simulink model "bd_par_auto2"  (Simulink 4.1.1)
settings: Solver=ode1  SolverMode=SingleTasking  StartTime=0.0  StopTime=max(cyc_mph(:,1))  FixedStep=1  MaxStep=1  RelTol=1e-3  AbsTol=1e-3
undefined symbols (not defined in the file): air_cp, amb_tmp, cs_charge_deplete_bool, cs_charge_trq, cs_electric_decel_spd, cs_electric_launch_spd_hi, cs_electric_launch_spd_lo, cs_hi_soc, cs_lo_soc, cs_min_trq_frac, cs_off_trq_frac, cyc_avg_time, cyc_cargo_mass, cyc_elevation_init, cyc_filter_bool, cyc_grade, cyc_mph, enable_stop, ess_cap_scale, ess_coulombic_eff, ess_init_soc, ess_max_ah_cap, ess_max_volts, ess_min_volts, ess_mod_airflow, ess_mod_cp, ess_mod_init_tmp, ess_module_mass, ess_module_num, ess_on, ess_res_scale_coef, ess_res_scale_fun, ess_set_tmp, ess_th_calc, ess_th_res_off, ess_th_res_on, ess_tmp, ess_voc, ex_calc, fc_ct_trq, fc_emis, fc_inertia, fc_map_spd, fc_max_trq, fc_on, fc_spd_scale, fc_trq_scale, fc_tstat, fd_inertia, fd_loss, fd_ratio, gb_dnshift_load, gb_dnshift_spd, gb_gears_num, gb_inertia, gb_num_init, gb_ratio, gb_shift_delay, gb_spd_scale, gb_trq_scale ... (+56)
libraries: lib_wheel2 x12, lib_accessory2 x3, lib_etc x2, lib_drive_cycle2 x1, lib_interactive x1, lib_drive_cycle x1, lib_exhaust x1, lib_fuel_converter3 x1
(part 3 of 18)

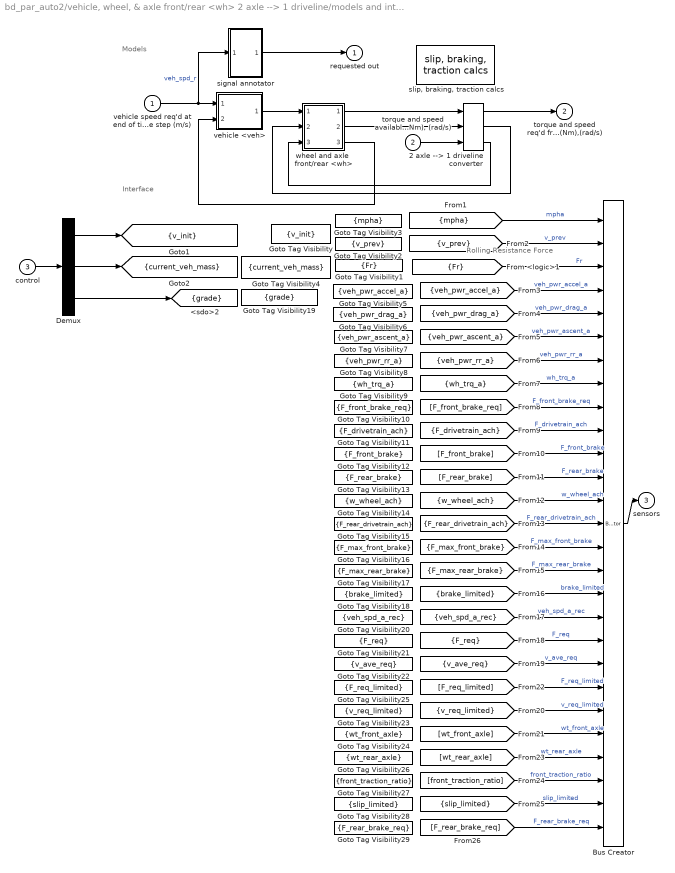
== system bd_par_auto2/vehicle, wheel, & axle front/rear <wh> 2 axle --> 1 driveline/models and interface ==
  note: Interface
  note: Models
  note: Rolling Resistance Force
  vehicle speed req'd at end of time step (m/s) : Inport  Port=1  LatchInput=off
  "torque and speed available from drivetrain into axles (Nm), (rad/s)" : Inport  Port=2  LatchInput=off
  control : Inport  Port=3  LatchInput=off
  2 axle --> 1 driveline converter : lib_wheel2/Submodels/2 axle --> 1 driveline converter
      settings: RTWFcnNameOpts=Auto  RTWFileNameOpts=Auto
  Bus Creator : BusCreator  Inputs=27
  Demux : Demux  Outputs=3  BusSelectionMode=off
  Goto Tag Visibility : GotoTagVisibility  GotoTag=v_init
  Goto Tag Visibility1 : GotoTagVisibility  GotoTag=Fr
  Goto Tag Visibility10 : GotoTagVisibility  GotoTag=F_front_brake_req
  Goto Tag Visibility11 : GotoTagVisibility  GotoTag=F_drivetrain_ach
  Goto Tag Visibility12 : GotoTagVisibility  GotoTag=F_front_brake
  Goto Tag Visibility13 : GotoTagVisibility  GotoTag=F_rear_brake
  Goto Tag Visibility14 : GotoTagVisibility  GotoTag=w_wheel_ach
  Goto Tag Visibility15 : GotoTagVisibility  GotoTag=F_rear_drivetrain_ach
  Goto Tag Visibility16 : GotoTagVisibility  GotoTag=F_max_front_brake
  Goto Tag Visibility17 : GotoTagVisibility  GotoTag=F_max_rear_brake
  Goto Tag Visibility18 : GotoTagVisibility  GotoTag=brake_limited
  Goto Tag Visibility19 : GotoTagVisibility  GotoTag=grade
  Goto Tag Visibility2 : GotoTagVisibility  GotoTag=v_prev
  Goto Tag Visibility20 : GotoTagVisibility  GotoTag=veh_spd_a_rec
  Goto Tag Visibility21 : GotoTagVisibility  GotoTag=F_req
  Goto Tag Visibility22 : GotoTagVisibility  GotoTag=v_ave_req
  Goto Tag Visibility23 : GotoTagVisibility  GotoTag=v_req_limited
  Goto Tag Visibility24 : GotoTagVisibility  GotoTag=wt_front_axle
  Goto Tag Visibility25 : GotoTagVisibility  GotoTag=F_req_limited
  Goto Tag Visibility26 : GotoTagVisibility  GotoTag=wt_rear_axle
  Goto Tag Visibility27 : GotoTagVisibility  GotoTag=front_traction_ratio
  Goto Tag Visibility28 : GotoTagVisibility  GotoTag=slip_limited
  Goto Tag Visibility29 : GotoTagVisibility  GotoTag=F_rear_brake_req
  Goto Tag Visibility3 : GotoTagVisibility  GotoTag=mpha
  Goto Tag Visibility4 : GotoTagVisibility  GotoTag=current_veh_mass
  Goto Tag Visibility5 : GotoTagVisibility  GotoTag=veh_pwr_accel_a
  Goto Tag Visibility6 : GotoTagVisibility  GotoTag=veh_pwr_drag_a
  Goto Tag Visibility7 : GotoTagVisibility  GotoTag=veh_pwr_ascent_a
  Goto Tag Visibility8 : GotoTagVisibility  GotoTag=veh_pwr_rr_a
  Goto Tag Visibility9 : GotoTagVisibility  GotoTag=wh_trq_a
  signal annotator : Subsystem
      settings: RTWFcnNameOpts=Auto  RTWFileNameOpts=Auto
  "slip, braking, traction calcs" : lib_wheel2/vehicle, wheel, & axle front//rear <wh>/models and interface/slip, braking, traction calcs
      link override config traction control: BlockChoice=traction control 2 axle
      settings: RTWFcnNameOpts=Auto  RTWFileNameOpts=Auto
  vehicle <veh> : Subsystem
      settings: RTWFcnNameOpts=Auto  RTWFileNameOpts=Auto
      mask Display: image(imread('bdi_veh.jpg'))
  wheel and axle  front/rear <wh> : Subsystem
      settings: RTWFcnNameOpts=Auto  RTWFileNameOpts=Auto
      mask Display: image(imread('bdi_wh.jpg'))
  requested out : Outport  Port=1  InitialOutput=0
  torque and speed req'd from drivetrain into axles (Nm),(rad/s) : Outport  Port=2  InitialOutput=0
  sensors : Outport  Port=3  InitialOutput=0
  tag scope: current_veh_mass=scoped, grade=scoped, v_init=scoped
  wires:
  signal annotator/1(Out1) -> requested out/1
  [F_rear_brake_req] -> Bus Creator/27  "F_rear_brake_req"
  [slip_limited] -> Bus Creator/26  "slip_limited"
  2 axle --> 1 driveline converter/1 -> torque and speed req'd from drivetrain into axles (Nm),(rad/s)/1
  2 axle --> 1 driveline converter/3 -> wheel and axle  front/rear <wh>/3("torque and speed available from drivetrain into rear axle (Nm), (rad/s)")
  2 axle --> 1 driveline converter/2 -> wheel and axle  front/rear <wh>/2("torque and speed available from drivetrain into front axle (Nm), (rad/s)")
  "torque and speed available from drivetrain into axles (Nm), (rad/s)"/1 -> 2 axle --> 1 driveline converter/3
  [front_traction_ratio] -> Bus Creator/25  "front_traction_ratio"
  [wt_rear_axle] -> Bus Creator/24  "wt_rear_axle"
  [wt_front_axle] -> Bus Creator/23  "wt_front_axle"
  [v_req_limited] -> Bus Creator/22  "v_req_limited"
  [F_req_limited] -> Bus Creator/21  "F_req_limited"
  [v_ave_req] -> Bus Creator/20  "v_ave_req"
  [F_req] -> Bus Creator/19  "F_req"
  [veh_spd_a_rec] -> Bus Creator/18  "veh_spd_a_rec"
  [brake_limited] -> Bus Creator/17  "brake_limited"
  [F_max_rear_brake] -> Bus Creator/16  "F_max_rear_brake"
  [F_max_front_brake] -> Bus Creator/15  "F_max_front_brake"
  [F_rear_drivetrain_ach] -> Bus Creator/14  "F_rear_drivetrain_ach"
  [w_wheel_ach] -> Bus Creator/13  "w_wheel_ach"
  [F_rear_brake] -> Bus Creator/12  "F_rear_brake"
  [F_front_brake] -> Bus Creator/11  "F_front_brake"
  [F_drivetrain_ach] -> Bus Creator/10  "F_drivetrain_ach"
  [F_front_brake_req] -> Bus Creator/9  "F_front_brake_req"
  [wh_trq_a] -> Bus Creator/8  "wh_trq_a"
  [veh_pwr_rr_a] -> Bus Creator/7  "veh_pwr_rr_a"
  [veh_pwr_ascent_a] -> Bus Creator/6  "veh_pwr_ascent_a"
  [veh_pwr_drag_a] -> Bus Creator/5  "veh_pwr_drag_a"
  [veh_pwr_accel_a] -> Bus Creator/4  "veh_pwr_accel_a"
  [v_prev] -> Bus Creator/2  "v_prev"
  [mpha] -> Bus Creator/1  "mpha"
  Bus Creator/1 -> sensors/1
  [Fr] -> Bus Creator/3  "Fr"
  Demux/3 -> [grade]
  Demux/2 -> [current_veh_mass]
  Demux/1 -> [v_init]
  control/1 -> Demux/1
  wheel and axle  front/rear <wh>/2(torque and speed req'd from drivetrain into rear axle (Nm),(rad/s)) -> 2 axle --> 1 driveline converter/2
  wheel and axle  front/rear <wh>/1(torque and speed req'd from drivetrain into front axle (Nm),(rad/s)) -> 2 axle --> 1 driveline converter/1
  wheel and axle  front/rear <wh>/3(tractive force and linear speed  achievable) -> vehicle <veh>/2(tractive force and linear speed achievable (N))
  vehicle <veh>/1("tractive force and speed required of tire and wheel (N), (m/s)") -> wheel and axle  front/rear <wh>/1("tractive force and speed req'd of tire/road interface (N), (m/s)")
  vehicle speed req'd at end of time step (m/s)/1 -> vehicle <veh>/1(vehicle speed req'd at end of time step (m/s)), signal annotator/1(veh_spd_r)  "veh_spd_r"

== system bd_par_auto2/<cs> control strategy/Automatic Transmission  Control/gearbox control for automatic transmission ==
  "eta_gb, t=(i-1)" : Inport  Port=1  LatchInput=off
  T_gb_out : Inport  Port=2  LatchInput=off
  w_gb_out : Inport  Port=3  LatchInput=off
  slip_limited : Inport  Port=4  LatchInput=off
  Goto Tag Visibility10 : GotoTagVisibility  GotoTag=gear_number
  Goto Tag Visibility11 : GotoTagVisibility  GotoTag=shifting
  Goto Tag Visibility12 : GotoTagVisibility  GotoTag=gear_ratio
  Goto Tag Visibility13 : GotoTagVisibility  GotoTag=locked_up
  Goto Tag Visibility6 : GotoTagVisibility  GotoTag=T_gb_out
  Goto Tag Visibility7 : GotoTagVisibility  GotoTag=w_gb_out
  Goto Tag Visibility8 : GotoTagVisibility  GotoTag=eta_gb
  Goto Tag Visibility9 : GotoTagVisibility  GotoTag=slip_limited
  gearbox control for use w/ AT : Subsystem
      settings: RTWFcnNameOpts=Auto  RTWFileNameOpts=Auto
  gear ratio : Outport  Port=1  InitialOutput=0
  shifting : Outport  Port=2  InitialOutput=0
  gear number : Outport  Port=3  InitialOutput=0
  locked_up : Outport  Port=4  InitialOutput=0
  tag scope: T_gb_out=scoped, eta_gb=scoped, gear_number=scoped, gear_ratio=scoped, locked_up=scoped, shifting=scoped, slip_limited=scoped, w_gb_out=scoped
  wires:
  T_gb_out/1 -> [T_gb_out]
  w_gb_out/1 -> [w_gb_out]
  [gear_number] -> gear number/1
  [shifting] -> shifting/1
  [gear_ratio] -> gear ratio/1
  slip_limited/1 -> [slip_limited]
  "eta_gb, t=(i-1)"/1 -> [eta_gb]
  [slip_limited] -> gearbox control for use w/ AT/4(tires are at traction limit)
  [w_gb_out] -> gearbox control for use w/ AT/3(gb_spd_out_r)
  [T_gb_out] -> gearbox control for use w/ AT/2(gb_trq_out_r)
  [eta_gb] -> gearbox control for use w/ AT/1(eta_gb)
  [locked_up] -> locked_up/1
  gearbox control for use w/ AT/1(gear ratio) -> [gear_ratio]
  gearbox control for use w/ AT/2(shifting) -> [shifting]
  gearbox control for use w/ AT/3(gear number) -> [gear_number]
  gearbox control for use w/ AT/4(locked up) -> [locked_up]

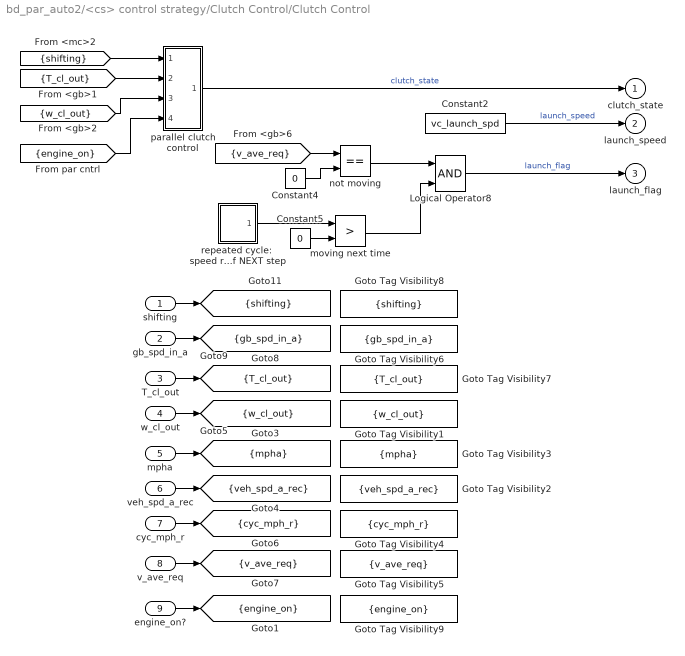
== system bd_par_auto2/<cs> control strategy/Clutch Control/Clutch Control ==
  shifting : Inport  Port=1  LatchInput=off
  gb_spd_in_a : Inport  Port=2  LatchInput=off
  T_cl_out : Inport  Port=3  LatchInput=off
  w_cl_out : Inport  Port=4  LatchInput=off
  mpha : Inport  Port=5  LatchInput=off
  veh_spd_a_rec : Inport  Port=6  LatchInput=off
  cyc_mph_r : Inport  Port=7  LatchInput=off
  v_ave_req : Inport  Port=8  LatchInput=off
  engine_on? : Inport  Port=9  LatchInput=off
  Constant2 : Constant  Value=vc_launch_spd
  Constant4 : Constant  Value=0
  Constant5 : Constant  Value=0
  Goto Tag Visibility1 : GotoTagVisibility  GotoTag=w_cl_out
  Goto Tag Visibility2 : GotoTagVisibility  GotoTag=veh_spd_a_rec
  Goto Tag Visibility3 : GotoTagVisibility  GotoTag=mpha
  Goto Tag Visibility4 : GotoTagVisibility  GotoTag=cyc_mph_r
  Goto Tag Visibility5 : GotoTagVisibility  GotoTag=v_ave_req
  Goto Tag Visibility6 : GotoTagVisibility  GotoTag=gb_spd_in_a
  Goto Tag Visibility7 : GotoTagVisibility  GotoTag=T_cl_out
  Goto Tag Visibility8 : GotoTagVisibility  GotoTag=shifting
  Goto Tag Visibility9 : GotoTagVisibility  GotoTag=engine_on
  Logical Operator8 : Logic  Operator=AND  Inputs=2
  moving next time : RelationalOperator  Operator=>
  not moving : RelationalOperator  Operator===
  parallel clutch control : Subsystem
      settings: RTWFcnNameOpts=Auto  RTWFileNameOpts=Auto
  repeated cycle:  speed required at end of NEXT step : Subsystem  mask(Forward looking repeating table){t=cyc_mph(:,1), y=cyc_mph(:,2)}
      mask prompts: t "Time values:"; y "Output values:"
      mask help:
      | Forward looking repeating table.
      | Enter values of time and output for first cycle.
      mask init:
      | period = max(t);
      settings: RTWFcnNameOpts=Auto  RTWFileNameOpts=Auto
      mask Help: Repeats cycle given in table with a one time step forward offset. Time values should be monotonically increasing.
  clutch_state : Outport  Port=1  InitialOutput=0
  launch_speed : Outport  Port=2  InitialOutput=0
  launch_flag : Outport  Port=3  InitialOutput=0
  tag scope: T_cl_out=scoped, cyc_mph_r=scoped, engine_on=scoped, gb_spd_in_a=scoped, mpha=scoped, shifting=scoped, v_ave_req=scoped, veh_spd_a_rec=scoped, w_cl_out=scoped
  wires:
  veh_spd_a_rec/1 -> [veh_spd_a_rec]
  T_cl_out/1 -> [T_cl_out]
  shifting/1 -> [shifting]
  gb_spd_in_a/1 -> [gb_spd_in_a]
  v_ave_req/1 -> [v_ave_req]
  cyc_mph_r/1 -> [cyc_mph_r]
  mpha/1 -> [mpha]
  w_cl_out/1 -> [w_cl_out]
  Constant2/1 -> launch_speed/1  "launch_speed"
  not moving/1 -> Logical Operator8/1
  Logical Operator8/1 -> launch_flag/1  "launch_flag"
  Constant4/1 -> not moving/2
  [v_ave_req] -> not moving/1
  repeated cycle:  speed required at end of NEXT step/1(out_1) -> moving next time/1
  Constant5/1 -> moving next time/2
  moving next time/1 -> Logical Operator8/2
  [engine_on] -> parallel clutch control/4(engine on)
  [T_cl_out] -> parallel clutch control/2(gb_trq_in_r)
  [w_cl_out] -> parallel clutch control/3(gb_spd_in_r)
  [shifting] -> parallel clutch control/1(shifting)
  parallel clutch control/1(clutch state) -> clutch_state/1  "clutch_state"
  engine_on?/1 -> [engine_on]

== system bd_par_auto2/<cs> control strategy/Electrical Accessories/electrical accessory controller ==
  electrical accessories on? : Inport  Port=1  LatchInput=off
  F_req in : Inport  Port=2  LatchInput=off
  key_on in : Inport  Port=3  LatchInput=off
  engine_on in : Inport  Port=4  LatchInput=off
  acc_on : Outport  Port=1  InitialOutput=0
  F_req : Outport  Port=2  InitialOutput=0
  key_on : Outport  Port=3  InitialOutput=0
  engine_on : Outport  Port=4  InitialOutput=0
  wires:
  electrical accessories on?/1 -> acc_on/1  "acc_on"
  engine_on in/1 -> engine_on/1  "engine_on"
  F_req in/1 -> F_req/1  "F_req"
  key_on in/1 -> key_on/1  "key_on"

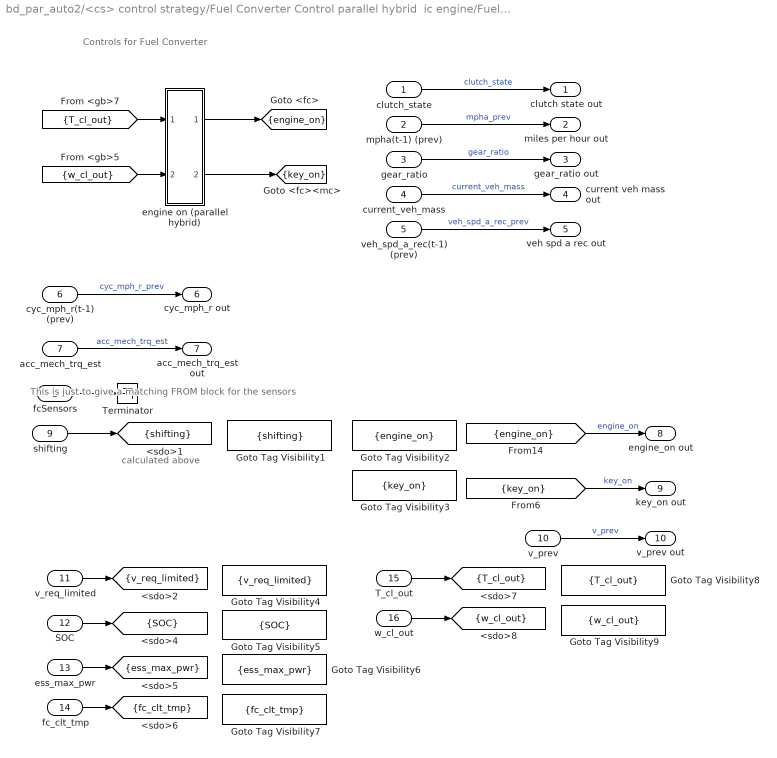
== system bd_par_auto2/<cs> control strategy/Fuel Converter Control parallel hybrid  ic engine/Fuel Converter Control ==
  note: Controls for Fuel Converter
  note: This is just to give a matching FROM block for the sensors
  note: calculated above
  clutch_state : Inport  Port=1  LatchInput=off
  mpha(t-1) (prev) : Inport  Port=2  LatchInput=off
  gear_ratio : Inport  Port=3  LatchInput=off
  current_veh_mass : Inport  Port=4  LatchInput=off
  veh_spd_a_rec(t-1) (prev) : Inport  Port=5  LatchInput=off
  cyc_mph_r(t-1) (prev) : Inport  Port=6  LatchInput=off
  acc_mech_trq_est : Inport  Port=7  LatchInput=off
  fcSensors : Inport  Port=8  LatchInput=off
  shifting : Inport  Port=9  LatchInput=off
  v_prev : Inport  Port=10  LatchInput=off
  v_req_limited : Inport  Port=11  LatchInput=off
  SOC : Inport  Port=12  LatchInput=off
  ess_max_pwr : Inport  Port=13  LatchInput=off
  fc_clt_tmp : Inport  Port=14  LatchInput=off
  T_cl_out : Inport  Port=15  LatchInput=off
  w_cl_out : Inport  Port=16  LatchInput=off
  Goto Tag Visibility1 : GotoTagVisibility  GotoTag=shifting
  Goto Tag Visibility2 : GotoTagVisibility  GotoTag=engine_on
  Goto Tag Visibility3 : GotoTagVisibility  GotoTag=key_on
  Goto Tag Visibility4 : GotoTagVisibility  GotoTag=v_req_limited
  Goto Tag Visibility5 : GotoTagVisibility  GotoTag=SOC
  Goto Tag Visibility6 : GotoTagVisibility  GotoTag=ess_max_pwr
  Goto Tag Visibility7 : GotoTagVisibility  GotoTag=fc_clt_tmp
  Goto Tag Visibility8 : GotoTagVisibility  GotoTag=T_cl_out
  Goto Tag Visibility9 : GotoTagVisibility  GotoTag=w_cl_out
  Terminator : Terminator
  engine on (parallel hybrid) : Subsystem
      settings: RTWFcnNameOpts=Auto  RTWFileNameOpts=Auto
  clutch state out : Outport  Port=1
  miles per hour out : Outport  Port=2
  gear_ratio out : Outport  Port=3
  current veh mass out : Outport  Port=4
  veh spd a rec out : Outport  Port=5
  cyc_mph_r out : Outport  Port=6
  acc_mech_trq_est out : Outport  Port=7
  engine_on out : Outport  Port=8
  key_on out : Outport  Port=9
  v_prev out : Outport  Port=10
  tag scope: SOC=scoped, T_cl_out=scoped, engine_on=scoped, ess_max_pwr=scoped, fc_clt_tmp=scoped, key_on=scoped, shifting=scoped, v_req_limited=scoped, w_cl_out=scoped
  wires:
  gear_ratio/1 -> gear_ratio out/1  "gear_ratio"
  fcSensors/1 -> Terminator/1
  shifting/1 -> [shifting]
  clutch_state/1 -> clutch state out/1  "clutch_state"
  mpha(t-1) (prev)/1 -> miles per hour out/1  "mpha_prev"
  current_veh_mass/1 -> current veh mass out/1  "current_veh_mass"
  veh_spd_a_rec(t-1) (prev)/1 -> veh spd a rec out/1  "veh_spd_a_rec_prev"
  cyc_mph_r(t-1) (prev)/1 -> cyc_mph_r out/1  "cyc_mph_r_prev"
  acc_mech_trq_est/1 -> acc_mech_trq_est out/1  "acc_mech_trq_est"
  v_prev/1 -> v_prev out/1  "v_prev"
  [engine_on] -> engine_on out/1  "engine_on"
  [key_on] -> key_on out/1  "key_on"
  engine on (parallel hybrid)/1(engine on) -> [engine_on]
  [T_cl_out] -> engine on (parallel hybrid)/1(trq req'd out of clutch (N*m))
  [w_cl_out] -> engine on (parallel hybrid)/2(spd req'd out of clutch (N*m))
  engine on (parallel hybrid)/2(key on) -> [key_on]
  v_req_limited/1 -> [v_req_limited]
  SOC/1 -> [SOC]
  ess_max_pwr/1 -> [ess_max_pwr]
  fc_clt_tmp/1 -> [fc_clt_tmp]
  T_cl_out/1 -> [T_cl_out]
  w_cl_out/1 -> [w_cl_out]

== system bd_par_auto2/<cs> control strategy/Hybrid  Engine Torque Modification Strategy/parallel auto hybrid torque control ==
  tm_spd_out_r : Inport  Port=1  LatchInput=off
  SOC : Inport  Port=2  LatchInput=off
  engine_on : Inport  Port=3  LatchInput=off
  chg trq req'd (Nm) : Subsystem
      settings: RTWFcnNameOpts=Auto  RTWFileNameOpts=Auto
  minimum trq (Nm) : Subsystem
      settings: RTWFcnNameOpts=Auto  RTWFileNameOpts=Auto
  tm_torqueMod : Outport  Port=1
  tm_torqueMin : Outport  Port=2
  tm_enable : Outport  Port=3
  wires:
  tm_spd_out_r/1 -> minimum trq (Nm)/1("spd req'd in (N*m, rad/s)")
  SOC/1 -> minimum trq (Nm)/2(SOC), chg trq req'd (Nm)/1(SOC)
  minimum trq (Nm)/1(minimum trq (N*m)) -> tm_torqueMin/1
  engine_on/1 -> tm_enable/1
  chg trq req'd (Nm)/1(add'l trq req'd (Nm)) -> tm_torqueMod/1

== system bd_par_auto2/<cs> control strategy/Mechanical Accessories/mechanical accessory controller ==
  accessory reference shaft speed : Inport  Port=1  LatchInput=off
  maximum accessory speed : Inport  Port=2  LatchInput=off
  minimum accessory speed : Inport  Port=3  LatchInput=off
  electrical accessories on? : Inport  Port=4  LatchInput=off
  Force required for vehicle motion : Inport  Port=5  LatchInput=off
  key on? : Inport  Port=6  LatchInput=off
  engine on? : Inport  Port=7  LatchInput=off
  Constant : Constant  Value=eps
  Logical Operator : Logic  Operator=AND  Inputs=2
  Relational Operator : RelationalOperator  Operator=>
  acc_on : Outport  Port=1  InitialOutput=0
  acc_mech_spd_r : Outport  Port=2  InitialOutput=0
  acc_mech_spd_a : Outport  Port=3  InitialOutput=0
  acc_max_spd : Outport  Port=4  InitialOutput=0
  acc_min_spd : Outport  Port=5  InitialOutput=0
  elec_acc_on_bool : Outport  Port=6  InitialOutput=0
  F_req : Outport  Port=7  InitialOutput=0
  key_on : Outport  Port=8  InitialOutput=0
  engine_on : Outport  Port=9  InitialOutput=0
  wires:
  accessory reference shaft speed/1 -> [acc_mech_spd_r], [acc_mech_spd_a]
  maximum accessory speed/1 -> [acc_max_spd]
  minimum accessory speed/1 -> [acc_min_spd]
  electrical accessories on?/1 -> [elec_acc_on_bool]
  Force required for vehicle motion/1 -> [F_req]
  key on?/1 -> [key_on]
  engine on?/1 -> [engine_on]
  [acc_mech_spd_r] -> Relational Operator/1
  Constant/1 -> Relational Operator/2
  [engine_on] -> Logical Operator/1
  Relational Operator/1 -> Logical Operator/2
  Logical Operator/1 -> [acc_on]
  [acc_on] -> acc_on/1  "acc_on"
  [engine_on] -> engine_on/1  "engine_on"
  [key_on] -> key_on/1  "key_on"
  [F_req] -> F_req/1  "F_req"
  [elec_acc_on_bool] -> elec_acc_on_bool/1  "elec_acc_on_bool"
  [acc_min_spd] -> acc_min_spd/1  "acc_min_spd"
  [acc_max_spd] -> acc_max_spd/1  "acc_max_spd"
  [acc_mech_spd_a] -> acc_mech_spd_a/1  "acc_mech_spd_a"
  [acc_mech_spd_r] -> acc_mech_spd_r/1  "acc_mech_spd_r"

== system bd_par_auto2/<cs> control strategy/Motor Controller/motor controller ==
  v_prev in : Inport  Port=1  LatchInput=off
  key_on in : Inport  Port=2  LatchInput=off
  veh_spd_a_rec_prev in : Inport  Port=3  LatchInput=off
  bus voltage previous : Inport  Port=4  LatchInput=off
  mpha_prev in : Inport  Port=5  LatchInput=off
  cyc_mph_r_prev in : Inport  Port=6  LatchInput=off
  current vehicle mass : Inport  Port=7  LatchInput=off
  shifting : Inport  Port=8  LatchInput=off
  mc_spd_init_est in : Inport  Port=9  LatchInput=off
  v_prev : Outport  Port=1
  key_on : Outport  Port=2
  veh_spd_a_rec_prev out : Outport  Port=3
  bus_voltage_prev : Outport  Port=4
  mpha_prev out : Outport  Port=5
  cyc_mph_r_prev : Outport  Port=6
  current_veh_mass : Outport  Port=7
  shifting out : Outport  Port=8
  mc_spd_init_est out : Outport  Port=9
  wires:
  bus voltage previous/1 -> bus_voltage_prev/1
  v_prev in/1 -> v_prev/1
  key_on in/1 -> key_on/1
  veh_spd_a_rec_prev in/1 -> veh_spd_a_rec_prev out/1
  mpha_prev in/1 -> mpha_prev out/1
  cyc_mph_r_prev in/1 -> cyc_mph_r_prev/1
  current vehicle mass/1 -> current_veh_mass/1
  shifting/1 -> shifting out/1
  mc_spd_init_est in/1 -> mc_spd_init_est out/1

== system bd_par_auto2/<cs> control strategy/Power Bus/power bus controller ==
  enable source two on power bus? : Inport  Port=1  LatchInput=off
  ess_on : Outport  Port=1
  wires:
  enable source two on power bus?/1 -> ess_on/1

== system bd_par_auto2/ACC MECH <accm>/mechanical accessory model and interface/Block NOTES ==

== system bd_par_auto2/ACC MECH <accm>/mechanical accessory model and interface/Mechanical Accessory model ==
  note: Reference Speed for speed dependant accessories
  note: Backward-Forward Models
  "requested shaft T and w, out to the driveline  (Nm ; rad/s; rad/s)" : Inport  Port=1  LatchInput=off
  "achieved shaft and belt T and w, in from the prime mover (Nm ; rad/s)" : Inport  Port=2  LatchInput=off
  Block NOTES : Subsystem
      settings: RTWFcnNameOpts=Auto  RTWFileNameOpts=Auto
      mask Display: disp('Block\nNOTES')
  Demux : Demux  Outputs=2  BusSelectionMode=off
  Demux1 : Demux  Outputs=2  BusSelectionMode=off
  Mux1 : Mux  Inputs=2
  Mux2 : Mux  Inputs=2
  backward model : Subsystem
      settings: RTWFcnNameOpts=Auto  RTWFileNameOpts=Auto
  f1 : Subsystem  TreatAsAtomicUnit=on  mask(enhancedToWorkspace){generalName=generalName, specificName=mech_pwr_a, logFlag=logFlag}
      mask prompts: generalName "General Name [char-evaluated]"; specificName "Specific Name [char-literal]"; logFlag "Enable flag (1=on,0=off)"
      mask help: A wrapper for the Simulink "To Workspace" block that allows you to evaluate the name of the variable to log to workspace. This is useful to avoid the double logging errors that occur when you pull in two library models that attempt to log to the same variable.
      mask init:
      | enhancedToWsMaker
      settings: CopyFcn=breakLinkCopyFcn  ParentCloseFcn=breakLinkParCloseFcn  RTWFcnNameOpts=Auto  RTWFileNameOpts=Auto
      mask Help:
      | <h2>Enhanced To Workspace Block</h2>
      | <h3>Parameters</h3>
      | <UL>
      | <li><b>General Name:</b> This is the more general name of the variable. Variables are saved to the workspace as <i>generalName_specificName</i>. Note that this is an evaluated variable. If you would like to type in the value directly, it must be surrounded with single quotes. Otherwise you can input the name of a variable containing a char string.</li>
      | <li><b>Specific Name:</b> This is the specific name of the variable. Note that this is input as a char literal (i.e., you don't need quotes).</li>
      | <li><b>Enable Flag:</b> This flag should have the value of 0 or 1. If 0, the variable will not be logged to the workspace. If 1, the variable will be logged. This is done so that variable logging can be turned off to improve speed.</li>
      | </ul>
      | <h3>Overview</h3>
      | <p>The enhanced to workspace block was put together to allow one to dynamically resolve variable names at run time in simulink. This is most powerful when used in conjunction with a masked subsystem to allow multiple instances of that masked subsytem to be used in the same model. The strategy is to set the generalName in the block mask which will allow the block to change the general name for all variable logging on the fly.
      | <h3>Helper Files</h3>
      | <p>Three m-files are required by the enhancedToWorkspace block. These files are located in the &lt; ADVISOR root &gt;/GUI directory :
      | <ul>
      | <li><i>enhancedToWsMaker.m</i> This file runs the mask initialization for the block</li>
      | <li><i>breakLinkCopyFcn.m</i> This file is used by the block callback when the simulink block is copied. It is necessary to break the link to the enhancedToWorkspace similar to the To Workspace block in order for it to be able to configure itself. (Try copying simulink's To Workspace block--it is impossible to make a link)</li>
      | <li><i>breakLinkParCloseFcn.m</i> This file is similar to the breakLinkCopyFcn and is used when a parent system is closed</li>
      | </ul>
      | <hr>
      | 
      | <p>Created 2003-Jan-21, Michael Patrick O'Keefe, NREL</p>
      | 
      | <!--
      | <VARDEF>
      | <H3>var_name</H3>
      | <UL>
      | <LI><B>data type</B> data type here</LI>
      | <LI><B>units</B> units here</LI>
      | <LI><B>vehicle type</B> vehicle type here</LI>
      | <LI><B>description</B> description here</LI>
      | </UL>
      | </VARDEF>
      | -->
      mask Display: disp([generalName,'_',specificName])
  f2 : Subsystem  TreatAsAtomicUnit=on  mask(enhancedToWorkspace){generalName=generalName, specificName=mech_trq_a, logFlag=logFlag}
      mask prompts: generalName "General Name [char-evaluated]"; specificName "Specific Name [char-literal]"; logFlag "Enable flag (1=on,0=off)"
      mask help: A wrapper for the Simulink "To Workspace" block that allows you to evaluate the name of the variable to log to workspace. This is useful to avoid the double logging errors that occur when you pull in two library models that attempt to log to the same variable.
      mask init:
      | enhancedToWsMaker
      settings: CopyFcn=breakLinkCopyFcn  ParentCloseFcn=breakLinkParCloseFcn  RTWFcnNameOpts=Auto  RTWFileNameOpts=Auto
      mask Help:
      | <h2>Enhanced To Workspace Block</h2>
      | <h3>Parameters</h3>
      | <UL>
      | <li><b>General Name:</b> This is the more general name of the variable. Variables are saved to the workspace as <i>generalName_specificName</i>. Note that this is an evaluated variable. If you would like to type in the value directly, it must be surrounded with single quotes. Otherwise you can input the name of a variable containing a char string.</li>
      | <li><b>Specific Name:</b> This is the specific name of the variable. Note that this is input as a char literal (i.e., you don't need quotes).</li>
      | <li><b>Enable Flag:</b> This flag should have the value of 0 or 1. If 0, the variable will not be logged to the workspace. If 1, the variable will be logged. This is done so that variable logging can be turned off to improve speed.</li>
      | </ul>
      | <h3>Overview</h3>
      | <p>The enhanced to workspace block was put together to allow one to dynamically resolve variable names at run time in simulink. This is most powerful when used in conjunction with a masked subsystem to allow multiple instances of that masked subsytem to be used in the same model. The strategy is to set the generalName in the block mask which will allow the block to change the general name for all variable logging on the fly.
      | <h3>Helper Files</h3>
      | <p>Three m-files are required by the enhancedToWorkspace block. These files are located in the &lt; ADVISOR root &gt;/GUI directory :
      | <ul>
      | <li><i>enhancedToWsMaker.m</i> This file runs the mask initialization for the block</li>
      | <li><i>breakLinkCopyFcn.m</i> This file is used by the block callback when the simulink block is copied. It is necessary to break the link to the enhancedToWorkspace similar to the To Workspace block in order for it to be able to configure itself. (Try copying simulink's To Workspace block--it is impossible to make a link)</li>
      | <li><i>breakLinkParCloseFcn.m</i> This file is similar to the breakLinkCopyFcn and is used when a parent system is closed</li>
      | </ul>
      | <hr>
      | 
      | <p>Created 2003-Jan-21, Michael Patrick O'Keefe, NREL</p>
      | 
      | <!--
      | <VARDEF>
      | <H3>var_name</H3>
      | <UL>
      | <LI><B>data type</B> data type here</LI>
      | <LI><B>units</B> units here</LI>
      | <LI><B>vehicle type</B> vehicle type here</LI>
      | <LI><B>description</B> description here</LI>
      | </UL>
      | </VARDEF>
      | -->
      mask Display: disp([generalName,'_',specificName])
  forward model : Subsystem
      settings: RTWFcnNameOpts=Auto  RTWFileNameOpts=Auto
  limit accessory mechanical speed achieved : lib_etc/saturation with inputs
      settings: RTWFcnNameOpts=Auto  RTWFileNameOpts=Auto
  limit accessory mechanical speed request : lib_etc/saturation with inputs
      settings: RTWFcnNameOpts=Auto  RTWFileNameOpts=Auto
  mechanical power logging : lib_accessory2/SubLibraries/mechanical power logging  eff=acc_mech_eff
  "requested shaft and belt T and w, in from the prime mover (Nm ; rad/s)" : Outport  Port=1
  "achieved shaft T and w, out to the driveline (Nm ; rad/s)" : Outport  Port=2
  tag scope: acc_mech_pwr_a=scoped, acc_mech_trq_a=scoped, w_APU_speed=scoped
  wires:
  [acc_min_spd] -> limit accessory mechanical speed achieved/3
  [acc_max_spd] -> limit accessory mechanical speed achieved/1
  [acc_mech_spd_a] -> limit accessory mechanical speed achieved/2
  limit accessory mechanical speed achieved/1 -> forward model/2(spd_in)
  [acc_min_spd] -> limit accessory mechanical speed request/3
  [acc_max_spd] -> limit accessory mechanical speed request/1
  limit accessory mechanical speed request/1 -> [w_APU_speed], backward model/2(spd_in)
  [acc_mech_spd_r] -> limit accessory mechanical speed request/2
  [acc_mech_trq_r] -> forward model/3(acc_trq_req)
  forward model/3(acc_mech_pwr_a) -> mechanical power logging/1, f1/1(In1), [acc_mech_pwr_a]
  forward model/2(acc_mech_trq_a) -> f2/1(In1), [acc_mech_trq_a]
  Mux2/1 -> "achieved shaft T and w, out to the driveline (Nm ; rad/s)"/1
  Mux1/1 -> "requested shaft and belt T and w, in from the prime mover (Nm ; rad/s)"/1
  "achieved shaft and belt T and w, in from the prime mover (Nm ; rad/s)"/1 -> Demux1/1
  "requested shaft T and w, out to the driveline  (Nm ; rad/s; rad/s)"/1 -> Demux/1
  Demux/1 -> backward model/1(trq1)  "trq out r"
  Demux/2 -> Mux1/2  "w shaft out r"
  backward model/1(trq2) -> Mux1/1  "trq in r"
  forward model/1(trq_out) -> Mux2/1
  Demux1/1 -> forward model/1(trq_in)  "trq in achieved from prime mover"
  Demux1/2 -> Mux2/2  "w shaft achieved by prime mover"

== system bd_par_auto2/ACC MECH <accm>/mechanical accessory model and interface/help ==

== system bd_par_auto2/ACC MECH <accm>/mechanical accessory model and interface/signal annotator ==
  In1 : Inport  Port=1  LatchInput=off
  Demux : Demux  Outputs=2  BusSelectionMode=off
  Mux : Mux  Inputs=2
  enhancedToWorkspace : Subsystem  TreatAsAtomicUnit=on  mask(enhancedToWorkspace){generalName=generalName, specificName=pre_acc_spd_out_r, logFlag=logFlag}
      mask prompts: generalName "General Name [char-evaluated]"; specificName "Specific Name [char-literal]"; logFlag "Enable flag (1=on,0=off)"
      mask help: A wrapper for the Simulink "To Workspace" block that allows you to evaluate the name of the variable to log to workspace. This is useful to avoid the double logging errors that occur when you pull in two library models that attempt to log to the same variable.
      mask init:
      | enhancedToWsMaker
      settings: CopyFcn=breakLinkCopyFcn  ParentCloseFcn=breakLinkParCloseFcn  RTWFcnNameOpts=Auto  RTWFileNameOpts=Auto
      mask Help:
      | <h2>Enhanced To Workspace Block</h2>
      | <h3>Parameters</h3>
      | <UL>
      | <li><b>General Name:</b> This is the more general name of the variable. Variables are saved to the workspace as <i>generalName_specificName</i>. Note that this is an evaluated variable. If you would like to type in the value directly, it must be surrounded with single quotes. Otherwise you can input the name of a variable containing a char string.</li>
      | <li><b>Specific Name:</b> This is the specific name of the variable. Note that this is input as a char literal (i.e., you don't need quotes).</li>
      | <li><b>Enable Flag:</b> This flag should have the value of 0 or 1. If 0, the variable will not be logged to the workspace. If 1, the variable will be logged. This is done so that variable logging can be turned off to improve speed.</li>
      | </ul>
      | <h3>Overview</h3>
      | <p>The enhanced to workspace block was put together to allow one to dynamically resolve variable names at run time in simulink. This is most powerful when used in conjunction with a masked subsystem to allow multiple instances of that masked subsytem to be used in the same model. The strategy is to set the generalName in the block mask which will allow the block to change the general name for all variable logging on the fly.
      | <h3>Helper Files</h3>
      | <p>Three m-files are required by the enhancedToWorkspace block. These files are located in the &lt; ADVISOR root &gt;/GUI directory :
      | <ul>
      | <li><i>enhancedToWsMaker.m</i> This file runs the mask initialization for the block</li>
      | <li><i>breakLinkCopyFcn.m</i> This file is used by the block callback when the simulink block is copied. It is necessary to break the link to the enhancedToWorkspace similar to the To Workspace block in order for it to be able to configure itself. (Try copying simulink's To Workspace block--it is impossible to make a link)</li>
      | <li><i>breakLinkParCloseFcn.m</i> This file is similar to the breakLinkCopyFcn and is used when a parent system is closed</li>
      | </ul>
      | <hr>
      | 
      | <p>Created 2003-Jan-21, Michael Patrick O'Keefe, NREL</p>
      | 
      | <!--
      | <VARDEF>
      | <H3>var_name</H3>
      | <UL>
      | <LI><B>data type</B> data type here</LI>
      | <LI><B>units</B> units here</LI>
      | <LI><B>vehicle type</B> vehicle type here</LI>
      | <LI><B>description</B> description here</LI>
      | </UL>
      | </VARDEF>
      | -->
      mask Display: disp([generalName,'_',specificName])
  enhancedToWorkspace1 : Subsystem  TreatAsAtomicUnit=on  mask(enhancedToWorkspace){generalName=generalName, specificName=pre_acc_trq_out_r, logFlag=logFlag}
      mask prompts: generalName "General Name [char-evaluated]"; specificName "Specific Name [char-literal]"; logFlag "Enable flag (1=on,0=off)"
      mask help: A wrapper for the Simulink "To Workspace" block that allows you to evaluate the name of the variable to log to workspace. This is useful to avoid the double logging errors that occur when you pull in two library models that attempt to log to the same variable.
      mask init:
      | enhancedToWsMaker
      settings: CopyFcn=breakLinkCopyFcn  ParentCloseFcn=breakLinkParCloseFcn  RTWFcnNameOpts=Auto  RTWFileNameOpts=Auto
      mask Help:
      | <h2>Enhanced To Workspace Block</h2>
      | <h3>Parameters</h3>
      | <UL>
      | <li><b>General Name:</b> This is the more general name of the variable. Variables are saved to the workspace as <i>generalName_specificName</i>. Note that this is an evaluated variable. If you would like to type in the value directly, it must be surrounded with single quotes. Otherwise you can input the name of a variable containing a char string.</li>
      | <li><b>Specific Name:</b> This is the specific name of the variable. Note that this is input as a char literal (i.e., you don't need quotes).</li>
      | <li><b>Enable Flag:</b> This flag should have the value of 0 or 1. If 0, the variable will not be logged to the workspace. If 1, the variable will be logged. This is done so that variable logging can be turned off to improve speed.</li>
      | </ul>
      | <h3>Overview</h3>
      | <p>The enhanced to workspace block was put together to allow one to dynamically resolve variable names at run time in simulink. This is most powerful when used in conjunction with a masked subsystem to allow multiple instances of that masked subsytem to be used in the same model. The strategy is to set the generalName in the block mask which will allow the block to change the general name for all variable logging on the fly.
      | <h3>Helper Files</h3>
      | <p>Three m-files are required by the enhancedToWorkspace block. These files are located in the &lt; ADVISOR root &gt;/GUI directory :
      | <ul>
      | <li><i>enhancedToWsMaker.m</i> This file runs the mask initialization for the block</li>
      | <li><i>breakLinkCopyFcn.m</i> This file is used by the block callback when the simulink block is copied. It is necessary to break the link to the enhancedToWorkspace similar to the To Workspace block in order for it to be able to configure itself. (Try copying simulink's To Workspace block--it is impossible to make a link)</li>
      | <li><i>breakLinkParCloseFcn.m</i> This file is similar to the breakLinkCopyFcn and is used when a parent system is closed</li>
      | </ul>
      | <hr>
      | 
      | <p>Created 2003-Jan-21, Michael Patrick O'Keefe, NREL</p>
      | 
      | <!--
      | <VARDEF>
      | <H3>var_name</H3>
      | <UL>
      | <LI><B>data type</B> data type here</LI>
      | <LI><B>units</B> units here</LI>
      | <LI><B>vehicle type</B> vehicle type here</LI>
      | <LI><B>description</B> description here</LI>
      | </UL>
      | </VARDEF>
      | -->
      mask Display: disp([generalName,'_',specificName])
  Out1 : Outport  Port=1
  wires:
  Mux/1 -> Out1/1
  Demux/2 -> Mux/2, enhancedToWorkspace/1(In1)  "macc_spd_out_r"
  Demux/1 -> Mux/1, enhancedToWorkspace1/1(In1)  "macc_trq_out_r"
  In1/1 -> Demux/1
